simulink library "NEARLib"  (R2022b)
settings: Solver=VariableStepAuto  StartTime=0.0  StopTime=10.0  RelTol=1e-3
values from neighbouring files (symbols this model uses):
  fsEQ = FsEQClass(near.front_peripheral_channel_count, near.frame_size/near.decimation_factor)    [NEARInit.m]
  hrEQ = HrEQClass(near.headrest_count, near.ann_sysin_channel_count,     near.frame_size/near.decimation_factor)    [NEARInit.m]
  NEAR_frame_size = 32    [NEARInit.m]
  NEAR_rear_channel_count = 3    [NEARInit.m]
libraries: HandyTextFile x2, BandsplitterCommon x1, FsEQLib x1, HrEQLib x1, PostmixLib x1, Router x1, UpmixerLib x1, VolMuteVNCALD x1
settings Model: Creator=ak1044356  LastModifiedBy=sa1045272
settings SolverCC: AlgebraicLoopSolver=TrustRegion
settings DebuggingCC: UnconnectedInputMsg=warning  UnconnectedOutputMsg=warning  UnconnectedLineMsg=warning  SFMachineParentedDataDiag=warning  ArithmeticOperatorsInVariantConditions=warning
settings ModelReferenceCC: EnableRefExpFcnMdlSchedulingChecks=on
settings SFSimCC: CustomCodeUndefinedFunction=UseInterfaceOnly

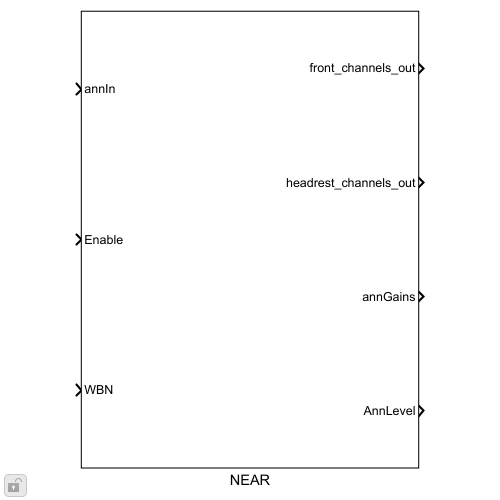
[thumbnail: Simulink's stored preview of the top-level diagram]
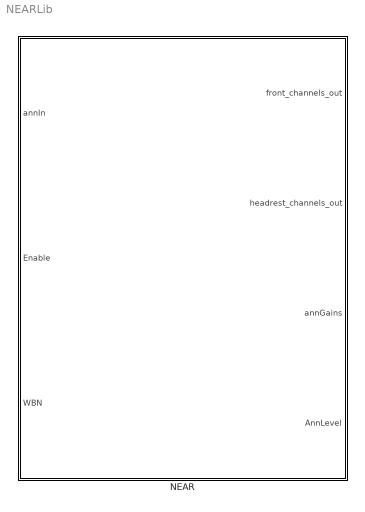
== system NEARLib ==
  NEAR : Subsystem

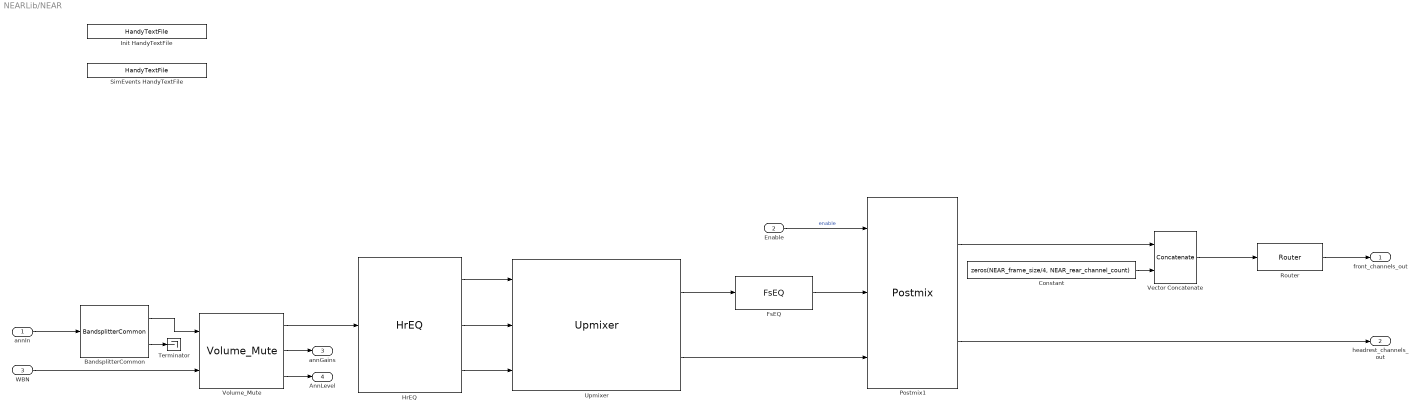
== system NEARLib/NEAR ==
  annIn : Inport  OutDataTypeStr=single
  Enable : Inport  Port=2
  WBN : Inport  Port=3
  BandsplitterCommon : BandsplitterCommon/BandsplitterCommon  Config=bandsplitter
  Constant : Constant  Value=zeros(NEAR_frame_size/4, NEAR_rear_channel_count)  OutDataTypeStr=single
  FsEQ : FsEQLib/FsEQ  Config=[fsEQ]
  HrEQ : HrEQLib/HrEQ  Config=[hrEQ]
  Init HandyTextFile : HandyTextFile/HandyTextFile  FileSuffix=Init.m  TheDefaultText=|
      | % Setup model parameters for each "Init" callback (e.g. update diagram)
      | sample_rate_in_hertz = 44100;
      | frame_size = 32;
      | sysin_channel_count = 2;
      | 
      | % setup simulation RTC data
      | run([ModelRootName() 'SimEvents.m']);
  Postmix1 : PostmixLib/Postmix  SystemSampleTime=-1  VariantActivationTime=update diagram  Latency=0  AutoFrameSizeCalculation=off
  Router : Router/Router  nInRouterMask=10  nOutRouterMask=6  outputMapDefaultRouterMask=[1 10 2 3 4 5]
  SimEvents HandyTextFile : HandyTextFile/HandyTextFile  FileSuffix=SimEvents.m  TheDefaultText=|
      | % Create RTC Simulation Object
      | RTC_SIM_OBJ = RTC_SimData();
      | 
      | % Add RTC requests for simulation
      | % RTC_SIM_OBJ.AddREQ( msg-name, time, arguments );
      | % e.g. RTC_SIM_OBJ.AddREQ( 'PreampVolumeSet', 0.5,  [0001, 255, 100,   0]);
  Terminator : Terminator
  Upmixer : UpmixerLib/Upmixer  SystemSampleTime=-1  VariantActivationTime=update diagram  Latency=0  AutoFrameSizeCalculation=off
  Vector Concatenate : Concatenate  Mode=Multidimensional array  ConcatenateDimension=2
  Volume_Mute : VolMuteVNCALD/Volume_Mute  vm=vm
  front_channels_out : Outport  VectorParamsAs1DForOutWhenUnconnected=off
  headrest_channels_out : Outport  Port=2  VectorParamsAs1DForOutWhenUnconnected=off
  annGains : Outport  Port=3
  AnnLevel : Outport  Port=4
  wires:
  Upmixer/1 -> FsEQ/1
  annIn/1 -> BandsplitterCommon/1
  Enable/1 -> Postmix1/1  "enable"
  Postmix1/1 -> Vector Concatenate/1
  BandsplitterCommon/1 -> Volume_Mute/1
  Volume_Mute/1 -> HrEQ/1
  Postmix1/2 -> headrest_channels_out/1
  Upmixer/2 -> Postmix1/3
  Vector Concatenate/1 -> Router/1
  Constant/1 -> Vector Concatenate/2
  FsEQ/1 -> Postmix1/2
  Volume_Mute/2 -> annGains/1
  WBN/1 -> Volume_Mute/2
  Router/1 -> front_channels_out/1
  Volume_Mute/3 -> AnnLevel/1
  HrEQ/1 -> Upmixer/1
  HrEQ/2 -> Upmixer/2
  HrEQ/3 -> Upmixer/3
  BandsplitterCommon/2 -> Terminator/1
